simulink model "lqr_control"  (R2019b)
settings: Solver=ode23  StartTime=0.0  StopTime=20  RelTol=1e-6
values from neighbouring files (symbols this model uses):
  A = [0,1,0,0 ... (first row only)    [dynamics.m]
  B = [0 ... (first row only)    [dynamics.m]
  C = [0,0,1,0]    [dynamics.m]
  D = zeros(size(C,1), size(B,2))    [dynamics.m]
  sample_time = 0.005    [dynamics.m]
  X_ref = [0,0,0.0,0]'    [dynamics.m]
undefined symbols (not defined in the file or in its folder): k
settings Model: Creator=lord-pradhan  LastModifiedBy=lord-pradhan

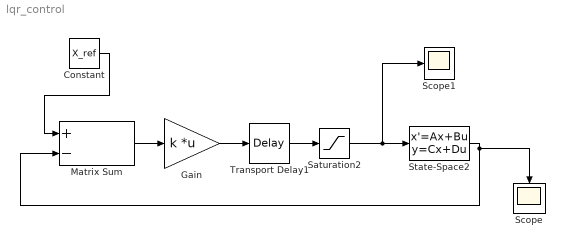
== system lqr_control ==
  Constant : Constant  Value=X_ref
  Gain : Gain  Gain=k  Multiplication=Matrix(K*u)
  Matrix Sum : Sum  Inputs=+-
  Saturation2 : Saturate  UpperLimit=8  LowerLimit=-8
  Scope : Scope
  Scope1 : Scope
  State-Space2 : StateSpace  A=A  B=B  C=C  D=D  InitialCondition=[0,0,0.11,0]  ContinuousStateAttributes="\"plant\""
  Transport Delay1 : TransportDelay  DelayTime=sample_time/2
  wires:
  Constant/1 -> Matrix Sum/1
  State-Space2/1 -> Scope/1, Matrix Sum/2
  Matrix Sum/1 -> Gain/1
  Gain/1 -> Transport Delay1/1
  Transport Delay1/1 -> Saturation2/1
  Saturation2/1 -> Scope1/1, State-Space2/1
